simulink model "non_linear_tank_Test_Dither"  (R2020a)
settings: Solver=VariableStepAuto  StartTime=0.0  StopTime=sim_time  RelTol=1e-3
undefined symbols (not defined in the file): k1, k2, p, r, sim_time, w, x1_0, x2_0
libraries: simulink x2, cstblocks x1
settings Model: Creator=jakelangton  LastModifiedBy=jakelangton
settings DataIOCC: Refine=5

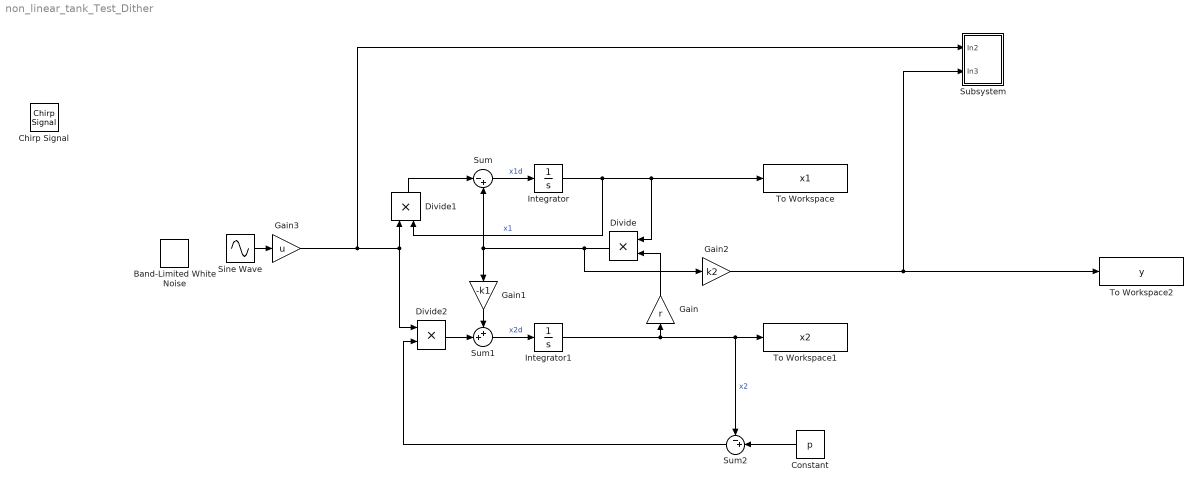
== system non_linear_tank_Test_Dither ==
  Band-Limited White Noise : simulink/Sources/Band-Limited White Noise  Cov=[1]  Ts=0.1  seed=[23341]
  Chirp Signal : simulink/Sources/Chirp Signal  f1=min_freq  T=sim_time  f2=max_freq
  Constant : Constant  Value=p
  Divide : Product  Inputs=**
  Divide1 : Product  Inputs=**
  Divide2 : Product  Inputs=**
  Gain : Gain  Gain=r
  Gain1 : Gain  Gain=-k1
  Gain2 : Gain  Gain=k2
  Gain3 : Gain  Gain=u
  Integrator : Integrator  InitialCondition=x1_0
  Integrator1 : Integrator  InitialCondition=x2_0
  Sine Wave : Sin  Amplitude=0.1  Frequency=w  SampleTime=0
  Subsystem : Subsystem
  Sum : Sum  Inputs=|-+
  Sum1 : Sum  Inputs=++|
  Sum2 : Sum  Inputs=-+|
  To Workspace : ToWorkspace  VariableName=x1  SaveFormat=Timeseries  SampleTime=-1
  To Workspace1 : ToWorkspace  VariableName=x2  SaveFormat=Timeseries  SampleTime=-1
  To Workspace2 : ToWorkspace  VariableName=y  SaveFormat=Timeseries  SampleTime=-1
  wires:
  Integrator1/1 -> Sum2/1, To Workspace1/1, Gain/1  "x2"
  Gain/1 -> Divide/2
  Integrator/1 -> Divide1/2, To Workspace/1, Divide/1  "x1"
  Sum/1 -> Integrator/1  "x1d"
  Divide/1 -> Gain2/1, Sum/2, Gain1/1
  Sum1/1 -> Integrator1/1  "x2d"
  Gain1/1 -> Sum1/1
  Divide1/1 -> Sum/1
  Gain2/1 -> Subsystem/2(In3), To Workspace2/1
  Sine Wave/1 -> Gain3/1
  Constant/1 -> Sum2/2
  Sum2/1 -> Divide2/2
  Divide2/1 -> Sum1/2
  Gain3/1 -> Subsystem/1(In2), Divide1/1, Divide2/1

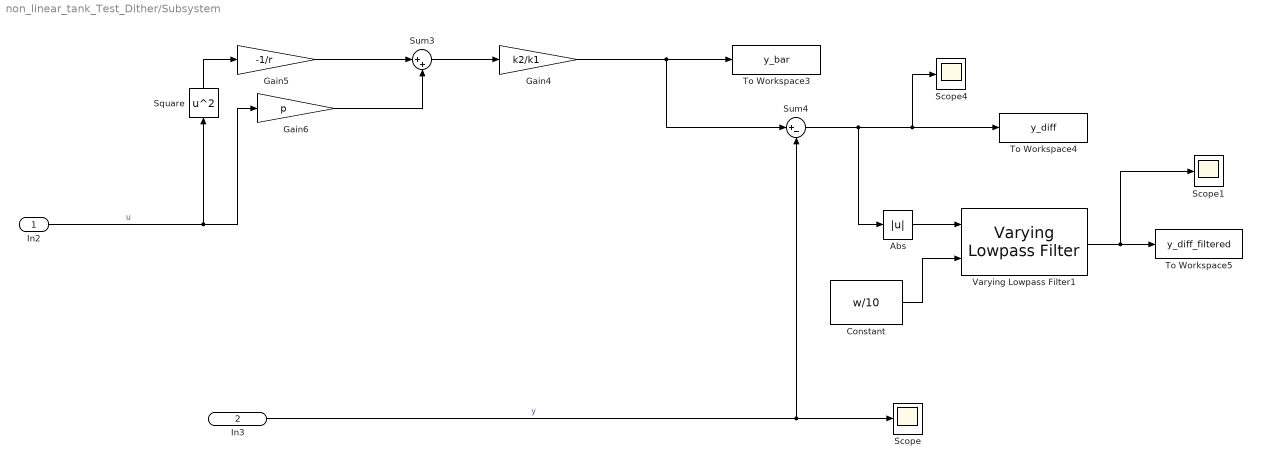
== system non_linear_tank_Test_Dither/Subsystem ==
  In2 : Inport
  In3 : Inport  Port=2
  Abs : Abs
  Constant : Constant  Value=w/10
  Gain4 : Gain  Gain=k2/k1
  Gain5 : Gain  Gain=-1/r
  Gain6 : Gain  Gain=p
  Scope : Scope
  Scope1 : Scope
  Scope4 : Scope
  Square : Math  Operator=square  SaturateOnIntegerOverflow=on
  Sum3 : Sum  Inputs=|++
  Sum4 : Sum  Inputs=|+-
  To Workspace3 : ToWorkspace  VariableName=y_bar  SaveFormat=Timeseries  SampleTime=-1
  To Workspace4 : ToWorkspace  VariableName=y_diff  SaveFormat=Timeseries  SampleTime=-1
  To Workspace5 : ToWorkspace  VariableName=y_diff_filtered  SaveFormat=Timeseries  SampleTime=-1
  Varying Lowpass Filter1 : cstblocks/Linear Parameter Varying/Varying Lowpass Filter  N=1
  wires:
  Square/1 -> Gain5/1
  In2/1 -> Square/1, Gain6/1  "u"
  Sum3/1 -> Gain4/1
  Gain6/1 -> Sum3/2
  Sum4/1 -> Abs/1, Scope4/1, To Workspace4/1
  In3/1 -> Scope/1, Sum4/2  "y"
  Gain5/1 -> Sum3/1
  Varying Lowpass Filter1/1 -> To Workspace5/1, Scope1/1
  Abs/1 -> Varying Lowpass Filter1/1
  Gain4/1 -> Sum4/1, To Workspace3/1
  Constant/1 -> Varying Lowpass Filter1/2
